simulink model "halfCarModel"  (R2016b)
settings: Solver=FixedStepAuto  StartTime=0.0  StopTime=1  FixedStep=.00005  RelTol=1e-3
settings Model: Creator=Devon  LastModifiedBy=Devon

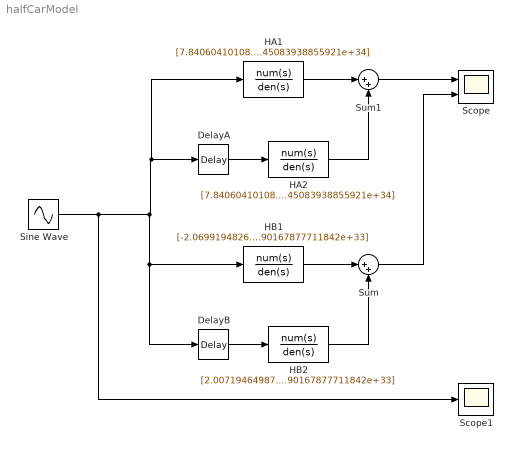
== system halfCarModel ==
  DelayA : TransportDelay  DelayTime=0.117117117117117
  DelayB : TransportDelay  DelayTime=0.117117117117117
  HA1 : TransferFcn  Numerator=[7.84060410108951e+29 3.70681037758283e+31 8.09326072199122e+32 7.14259391290688e+33]  Denominator=[8.92822413167542e+28 4.21887225471424e+30 1.21080571108626e+32 1.64394358415447e+33 1.45083938855921e+34]
  HA2 : TransferFcn  Numerator=[7.84060410108951e+29 3.71698061715107e+31 8.34617511955345e+32 7.36579997268522e+33]  Denominator=[8.92822413167542e+28 4.21887225471424e+30 1.21080571108626e+32 1.64394358415447e+33 1.45083938855921e+34]
  HB1 : TransferFcn  Numerator=[-2.06991948268763e+29 -7.3169027995277e+30 -1.26457198781113e+32 -1.1160302988917e+33]  Denominator=[1.78564482633508e+28 8.43774450942848e+29 2.42161142217252e+31 3.28788716830893e+32 2.90167877711842e+33]
  HB2 : TransferFcn  Numerator=[2.00719464987891e+29 7.04639378261576e+30 1.26457198781113e+32 1.1160302988917e+33]  Denominator=[1.78564482633508e+28 8.43774450942848e+29 2.42161142217252e+31 3.28788716830893e+32 2.90167877711842e+33]
  Scope : Scope  NumInputPorts=2
  Scope1 : Scope
  Sine Wave : Sin  Amplitude=0.015  Frequency=69.7  SampleTime=0
  Sum : Sum  Inputs=|++
  Sum1 : Sum  Inputs=|++
  wires:
  Sum1/1 -> Scope/1
  Sum/1 -> Scope/2
  HA1/1 -> Sum1/1
  HA2/1 -> Sum1/2
  HB1/1 -> Sum/1
  HB2/1 -> Sum/2
  DelayB/1 -> HB2/1
  Sine Wave/1 -> Scope1/1, HB1/1, DelayB/1, DelayA/1, HA1/1
  DelayA/1 -> HA2/1
